simulink model "Quadcopter_NMPC_2_Updated"  (R2021a)
settings: Solver=ode4  StartTime=0.0  StopTime=20  FixedStep=0.001  RelTol=1e-3
libraries: mpclib x1
settings Model: Creator=Hameed  LastModifiedBy=Hameed

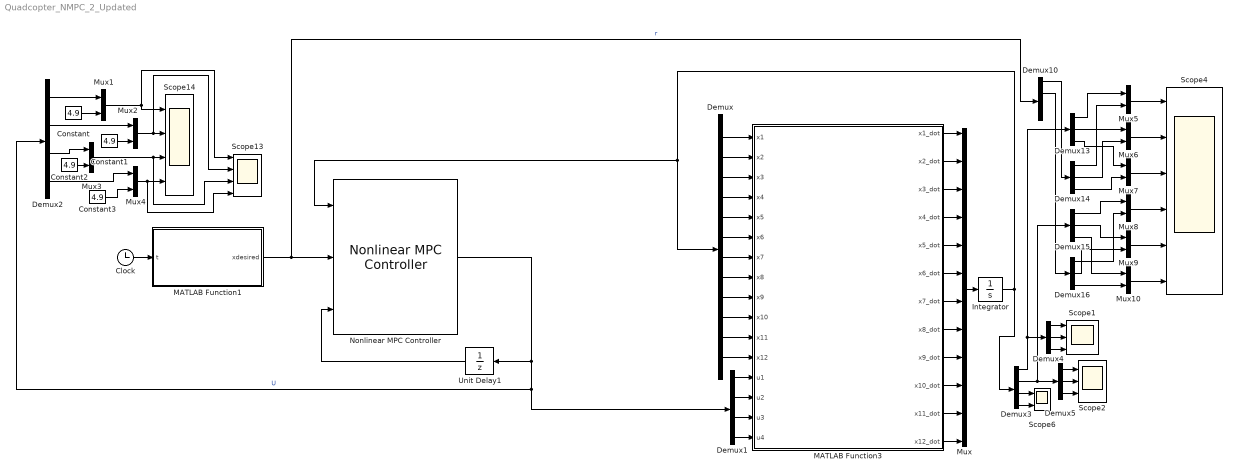
== system Quadcopter_NMPC_2_Updated ==
  Clock : Clock
  Constant{,1..3} (4 alike) : Constant  Value=4.9
  Demux : Demux  Outputs=12
  Demux{1..3,10} (4 alike) : Demux
  Demux{4..5,13..16} (6 alike) : Demux  Outputs=3
  Integrator : Integrator  InitialCondition=[7;-10;0;0;0;0;0;0;0;0;0;0]
  MATLAB Function1 : MATLAB Function  TreatAsAtomicUnit=on
  MATLAB Function3 : MATLAB Function  TreatAsAtomicUnit=on
  Mux : Mux  Inputs=12
  Mux{1..10} (10 alike) : Mux  Inputs=2
  Nonlinear MPC Controller : mpclib/Nonlinear MPC Controller  SCDEnableBlockLinearizationSpecification=on  nlmpcobj=nlobj  UseObjectTs=on  UseMEX=off  md_enabled=off  mvtarget_enabled=off  param_enabled=off  cost_enabled=off  mvseq_enabled=off  stateseq_enabled=off  ovseq_enabled=off  slack_enabled=off  status_enabled=off  ov_min=off  ov_max=off  mv_min=off  mv_max=off  mvrate_min=off  mvrate_max=off  state_min=off  state_max=off  ov_weight=off  mv_weight=off  mvrate_weight=off  ecr_weight=off  nlp_initialize=off
  Scope1 : Scope  NumInputPorts=3
  Scope13 : Scope  NumInputPorts=4
  Scope14 : Scope  NumInputPorts=4
  Scope2 : Scope  NumInputPorts=3
  Scope4 : Scope  NumInputPorts=6
  Scope6 : Scope  NumInputPorts=2
  Unit Delay1 : UnitDelay  InitialCondition=[4.9;4.9;4.9;4.9]  SampleTime=0.1  HasFrameUpgradeWarning=on
  wires:
  MATLAB Function3/7(x7_dot) -> Mux/7
  MATLAB Function3/8(x8_dot) -> Mux/8
  MATLAB Function3/5(x5_dot) -> Mux/5
  MATLAB Function3/4(x4_dot) -> Mux/4
  Nonlinear MPC Controller/1 -> Demux2/1, Demux1/1, Unit Delay1/1  "U"
  MATLAB Function3/6(x6_dot) -> Mux/6
  Integrator/1 -> Demux/1, Nonlinear MPC Controller/1, Demux3/1
  Mux/1 -> Integrator/1
  MATLAB Function3/12(x12_dot) -> Mux/12
  MATLAB Function3/3(x3_dot) -> Mux/3
  MATLAB Function3/1(x1_dot) -> Mux/1
  MATLAB Function1/1(xdesired) -> Demux10/1, Nonlinear MPC Controller/2  "r"
  MATLAB Function3/11(x11_dot) -> Mux/11
  MATLAB Function3/10(x10_dot) -> Mux/10
  Clock/1 -> MATLAB Function1/1(t)
  Unit Delay1/1 -> Nonlinear MPC Controller/3
  Demux2/1 -> Mux1/1
  Demux2/2 -> Mux2/1
  Demux2/3 -> Mux3/1
  Demux3/1 -> Demux4/1, Demux13/1
  Demux3/2 -> Demux15/1, Demux5/1
  Demux4/2 -> Scope1/2
  Demux4/1 -> Scope1/1
  Demux4/3 -> Scope1/3
  Demux5/3 -> Scope2/3
  Demux5/1 -> Scope2/1
  Demux5/2 -> Scope2/2
  Demux2/4 -> Mux4/1
  Constant/1 -> Mux1/2
  Constant1/1 -> Mux2/2
  Constant2/1 -> Mux3/2
  Constant3/1 -> Mux4/2
  Mux2/1 -> Scope13/2, Scope14/2
  Mux1/1 -> Scope14/1, Scope13/1
  Mux4/1 -> Scope13/4, Scope14/4
  Mux3/1 -> Scope13/3, Scope14/3
  Demux3/3 -> Scope6/1
  Demux3/4 -> Scope6/2
  Demux10/1 -> Demux14/1
  Demux10/2 -> Demux16/1
  Mux5/1 -> Scope4/1
  Mux6/1 -> Scope4/2
  Mux8/1 -> Scope4/4
  Mux9/1 -> Scope4/5
  Mux10/1 -> Scope4/6
  Demux13/1 -> Mux5/1
  Demux13/2 -> Mux6/1
  Demux13/3 -> Mux7/1
  Demux14/1 -> Mux5/2
  Demux14/2 -> Mux6/2
  Demux14/3 -> Mux7/2
  Demux15/1 -> Mux8/1
  Demux15/2 -> Mux9/1
  Demux15/3 -> Mux10/1
  Demux16/1 -> Mux8/2
  Demux16/2 -> Mux9/2
  Demux16/3 -> Mux10/2
  Mux7/1 -> Scope4/3
  MATLAB Function3/2(x2_dot) -> Mux/2
  MATLAB Function3/9(x9_dot) -> Mux/9
  Demux1/1 -> MATLAB Function3/13(u1)
  Demux1/2 -> MATLAB Function3/14(u2)
  Demux1/3 -> MATLAB Function3/15(u3)
  Demux1/4 -> MATLAB Function3/16(u4)
  Demux/1 -> MATLAB Function3/1(x1)
  Demux/2 -> MATLAB Function3/2(x2)
  Demux/3 -> MATLAB Function3/3(x3)
  Demux/4 -> MATLAB Function3/4(x4)
  Demux/5 -> MATLAB Function3/5(x5)
  Demux/6 -> MATLAB Function3/6(x6)
  Demux/7 -> MATLAB Function3/7(x7)
  Demux/8 -> MATLAB Function3/8(x8)
  Demux/9 -> MATLAB Function3/9(x9)
  Demux/10 -> MATLAB Function3/10(x10)
  Demux/11 -> MATLAB Function3/11(x11)
  Demux/12 -> MATLAB Function3/12(x12)

== matlab function Quadcopter_NMPC_2_Updated/MATLAB Function1 ==
  data: t input; xdesired output
function xdesired   = QuadrotorReferenceTrajectory( t )
% This function generates reference signal for nonlinear MPC controller
% used in the quadrotor path following example.

% Copyright 2019 The MathWorks, Inc.

%#codegen
x =6*sin(t/3);
y = -6*sin(t/3).*cos(t/3);
z = 6*cos(t/3);
%z = 10+zeros(1,length(t));
phi = zeros(1,length(t));
theta = zeros(1,length(t));
psi = zeros(1,length(t));
% phi = pi/6*sin(t/3);
% theta = -pi/3*sin(t/3).*cos(t/3);
% psi = pi*ones(1,length(t));
xdot = zeros(1,length(t));
ydot = zeros(1,length(t));
zdot = zeros(1,length(t));
phidot = zeros(1,length(t));
thetadot = zeros(1,length(t));
psidot = zeros(1,length(t));

xdesired = [x;y;z;phi;theta;psi;xdot;ydot;zdot;phidot;thetadot;psidot]';
end

== matlab function Quadcopter_NMPC_2_Updated/MATLAB Function3 ==
  data: x1 input; x1_dot output; x2 input; x3 input; x4 input; x5 input; x6 input; x7 input; x8 input; x9 input; x10 input; x11 input; x12 input; x2_dot output; x3_dot output; x4_dot output; x5_dot output; x6_dot output; x7_dot output; x8_dot output; x9_dot output; x10_dot output; x11_dot output; x12_dot output; u1 input; u2 input; u3 input; u4 input
function [x1_dot,x2_dot,x3_dot,x4_dot,x5_dot,x6_dot,x7_dot,x8_dot,x9_dot,x10_dot,x11_dot,x12_dot]= fcn(x1,x2,x3,x4,x5,x6,x7,x8,x9,x10,x11,x12,u1,u2,u3,u4)

Ixx= 1.2; 
Iyy= 1.2;
Izz= 2.3;
k=1;
%k = 1e-3;
L= 0.25;
m= 2;
km= 0.2;
%km = 0.5e-4;
g= 9.81;
gamma = km/k; 

Ixx = (1/12)*m*(0.2^2+0.2^2);
Iyy= (1/12)*m*(0.2^2+0.2^2);
Izz= (1/12)*m*(0.2^2+0.2^2);
I= [Ixx 0 0;0 Iyy 0;0 0 Izz];


%R-ZYX Euler
R = [cos(x5)*cos(x6), sin(x4)*sin(x5)*cos(x6)-cos(x4)*sin(x6), cos(x4)*sin(x5)*cos(x6)+sin(x4)*sin(x6);
     cos(x5)*sin(x6), sin(x4)*sin(x5)*sin(x6)+cos(x4)*cos(x6), cos(x4)*sin(x5)*sin(x6)-sin(x4)*cos(x6);
     -sin(x5), sin(x4)*cos(x5), cos(x4)*cos(x5)];


Q = [1 0 -sin(x5);
     0 cos(x4) cos(x5)*sin(x4);
     0 -sin(x4) cos(x5)*cos(x4)];

dQ = [0 0 -cos(x5);
      0 -sin(x4) -sin(x5)*sin(x4)+cos(x5)*cos(x4);
      0 -cos(x4) -sin(x5)*cos(x4)-cos(x5)*sin(x4)];


M = Q'.*I*Q;

ndot=[x10;x11;x12];
% s = Q*ndot;
% S = [0 -s(3) s(2);s(3) 0 -s(1);-s(2) s(1) 0];
% C = Q'.*S*I*Q + Q'.*I*dQ;
%%-------------------------------------------------------------------
C11=0;
C12=(Iyy-Izz)*(x11*cos(x4)*sin(x4)+x12*sin(x4)^2*cos(x5))+(Izz-Iyy)*x12*cos(x4)^2*cos(x5)-Ixx*x12*cos(x5);
C13=(Izz-Iyy)*(x12*cos(x4)*sin(x4)*cos(x5)^2);
C21=(Izz-Iyy)*(x11*cos(x4)*sin(x4)+x12*sin(x4)*cos(x5))+(Iyy-Izz)*x12*cos(x4)^2*cos(x5)+Ixx*x12*cos(x5);
C22=(Izz-Iyy)*x10*cos(x4)*sin(x4);
C23= -Ixx*x12*sin(x5)*cos(x5)+Iyy*x12*sin(x4)^2*sin(x5)*cos(x5)+ Izz*x12*cos(x4)^2*sin(x5)*cos(x5);
C31=(Iyy-Izz)*(x12*cos(x5)^2*sin(x4)*cos(x4))-Ixx*x11*cos(x5);
C32= (Izz-Iyy)*(x11*cos(x4)*sin(x4)*sin(x5)+x10*sin(x4)^2*cos(x5))+(Iyy-Izz)*x10*cos(x4)^2*cos(x5)+Ixx*x12*sin(x5)*cos(x5)-Iyy*x12*sin(x10)^2*sin(x5)*cos(x5)-Izz*x12*cos(x10)^2*sin(x5)*cos(x5);
C33=(Iyy-Izz)*x10*cos(x4)*sin(x4)*cos(x5)^2-Iyy*x11*sin(x4)^2*cos(x5)*sin(x5)-Izz*x11*cos(x4)^2*cos(x5)*sin(x5)+Ixx*x11*cos(x5)*sin(x5);
C=[C11 C12 C13;C21 C22 C23;C31 C32 C33];
%%---------------------------------------------------

% A = [ 1 1 1 1;
%       0  L 0 -L;
%      -L 0  L  0;
%      gamma -gamma gamma -gamma];
%  A = [ 0 0 0 0;
%       0 0 0 0;
%       1 1 1 1;
%       0  L 0 -L;
%      -L 0  L  0;
%      gamma -gamma gamma -gamma];


 %u = [uz;tx;ty;tz];
 u = [u1;u2;u3;u4];
%  th = pinv(A)*u;
%  %w = (th/k);         % actually it's omeega square
% w= sqrt(th/k);
% % %u=k*A*ws;
 


T = k*(u(1)+u(2)+u(3)+u(4));
%T = k*(w(1)^2+w(2)^2+w(3)^2+w(4)^2);

%tB= [L*k*(w(2)-w(4));L*k*(-w(1)+w(3));km*(w(1)-w(2)+w(3)-w(4))];
%tB= [L*k*(w(2)^2-w(4)^2);L*k*(-w(1)^2+w(3)^2);km*(w(1)^2-w(2)^2+w(3)^2-w(4)^2)];
tB= [L*k*(u2-u4);L*k*(-u1+u3);km*(u1-u2+u3-u4)];

%Jinv=inv(J)
%x789= g*[0;0;1]-R*[0;0;T]/m;


x789 = (1/m)*(-R*[0;0;T]+ m*g*[0;0;1]);
%x789 = (1/m)*(-k*R*A(1:3,:)*w+ m*g*[0;0;1] );


x101112 = inv(M)*(tB-C*ndot);
%x101112 = inv(M)*(Q'*tB-C*ndot);
%x101112= inv(M)*(Q'*k*A(4:6,:)*w -C*ndot );

x1_dot=x7;
x2_dot=x8;
x3_dot=x9;
x4_dot=x10;
x5_dot=x11;
x6_dot=x12;

x7_dot=x789(1);
x8_dot=x789(2);
x9_dot=x789(3);

x10_dot=x101112(1);
x11_dot=x101112(2);
x12_dot=x101112(3);


%%-----------------------------------------------------------------------------



% 
%references
% xd = 0; yd = 0; zd = -2;
% phid = pi/4.; thetad = pi/4.; psid = pi/4.;

%error signals
% ez = zd-x3;
% ephi = phid-x4;
% etheta = thetad-x5;
% epsi = psid-x6;

%controller
%u(1)  = 50*ez-60*dz+30*iez;
% u(1)  = 50*ez-60*dz;
% u(2)  = 1*ephi-2*dphi;
% u(3)  = 1*etheta-2*dtheta;
% u(4) = 1*epsi-2*dpsi;

% uz = -(50*ez-60*x9);
% tx = (1*ephi-2*x10);
% ty = (1*etheta-2*x11);
% tz = (1*epsi-2*x12);
